simulink model "examplePumpConst"  (R2016b)
settings: Solver=ode45  StartTime=0.0  StopTime=240  RelTol=1e-3  EnableMultiTasking=on
libraries: carnot x2
settings Model: Creator=drhf  LastModifiedBy=drhf
settings DataIOCC: LimitDataPoints=on  SaveFormat=Array
settings OptimizationCC: ExpressionDepthLimit=2147483647  LifeSpan=inf
settings DebuggingCC: UnderspecifiedInitializationDetection=Classic  MergeDetectMultiDrivingBlocksExec=none  SolverPrmCheckMsg=warning  StateNameClashWarn=warning  SFUnexpectedBacktrackingDiag=warning  SFNoUnconditionalDefaultTransitionDiag=warning  SFExecutionAtInitializationDiag=none
settings HardwareCC: ProdBitPerPointer=32  ProdBitPerSizeT=32  ProdBitPerPtrDiffT=32  ProdLargestAtomicFloat=None  ProdIntDivRoundTo=Undefined  ProdEndianess=Unspecified  ProdWordSize=32  ProdHWDeviceType=32-bit Generic
settings ModelReferenceCC: PropagateSignalLabelsOutOfModel=off
settings GRTTargetCC: TargetLangStandard=C89/C90 (ANSI)  GeneratePreprocessorConditionals=Disable all  CombineOutputUpdateFcns=off  GRTInterface=on
settings ConfigComp: CovMetricSettings=dw  CovHtmlReporting=on  CovSaveCumulativeToWorkspaceVar=on  CovSaveSingleToWorkspaceVar=on  CovExternalEMLEnable=off

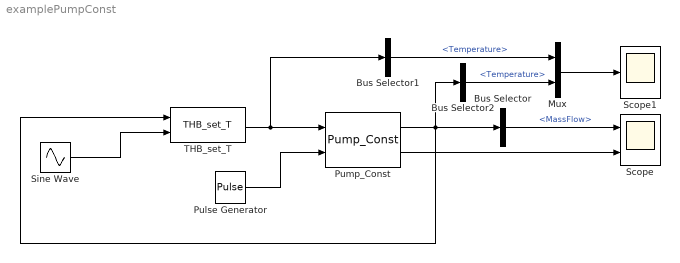
== system examplePumpConst ==
  Bus Selector : BusSelector  OutputSignals=MassFlow
  Bus Selector1 : BusSelector  OutputSignals=Temperature
  Bus Selector2 : BusSelector  OutputSignals=Temperature
  Mux : Mux  Inputs=2
  Pulse Generator : DiscretePulseGenerator  PulseType=Time based  Period=120  PulseWidth=50
  Pump_Const : carnot/Hydraulics/Pump_Const  mdotmax=1200/3600  dia=0.025  power=30  p0=3e5  fluid_id=Water  mix=0  mix2=0  mix3=0  UA=1  mcp=2000  tamb=20  cp_approx=4000
  Scope : Scope  NumInputPorts=2
  Scope1 : Scope
  Sine Wave : Sin  Amplitude=5  Bias=20  Frequency=2*pi/240  SampleTime=0
  THB_set_T : carnot/Source/Simple/THB_set_T
  wires:
  Pump_Const/1 -> THB_set_T/1, Bus Selector/1, Bus Selector2/1
  THB_set_T/1 -> Pump_Const/1, Bus Selector1/1
  Pulse Generator/1 -> Pump_Const/2
  Pump_Const/2 -> Scope/2
  Bus Selector/1 -> Scope/1  "<MassFlow>"
  Bus Selector1/1 -> Mux/1  "<Temperature>"
  Bus Selector2/1 -> Mux/2  "<Temperature>"
  Mux/1 -> Scope1/1
  Sine Wave/1 -> THB_set_T/2
